simulink subsystem "s0411_swing_fast2"  (R2019b)
settings: Solver=VariableStepAuto  StartTime=0.0  StopTime=10.0  RelTol=1e-3
settings Model: Creator=Student  LastModifiedBy=giaco

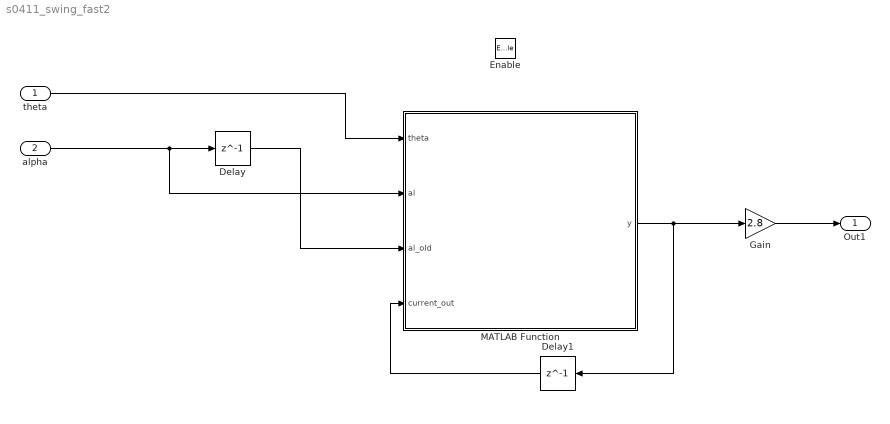
== system s0411_swing_fast2 ==
  theta : Inport
  alpha : Inport  Port=2
  Enable : EnablePort  StatesWhenEnabling=reset
  Delay : Delay  DelayLength=1  InitialCondition=0
  Delay1 : Delay  DelayLength=1  InitialCondition=1
  Gain : Gain  Gain=2.8
  MATLAB Function : MATLAB Function  TreatAsAtomicUnit=on
  Out1 : Outport
  wires:
  MATLAB Function/1(y) -> Gain/1, Delay1/1
  theta/1 -> MATLAB Function/1(theta)
  alpha/1 -> MATLAB Function/2(al), Delay/1
  Delay/1 -> MATLAB Function/3(al_old)
  Gain/1 -> Out1/1
  Delay1/1 -> MATLAB Function/4(current_out)

== matlab function s0411_swing_fast2/MATLAB Function ==
  data: theta input; y output; al input; al_old input; current_out input
function y = fcn(theta, al, al_old, current_out)

if al < al_old && current_out == 1
    
    signum = -1;
    
elseif al > al_old && current_out == -1
    
    signum = 1;
    
else
    signum = current_out;
    
end
    
if theta > pi/3 && signum == 1
    
    signum = -1;
    
elseif theta < -pi/3 && signum == -1
    
    signum = 1;
    
end

y = signum;
